simulink library "PS3Controller"  (R2026a)
settings: Solver=VariableStepAuto
settings Model: Creator=ebene  LastModifiedBy=ebene

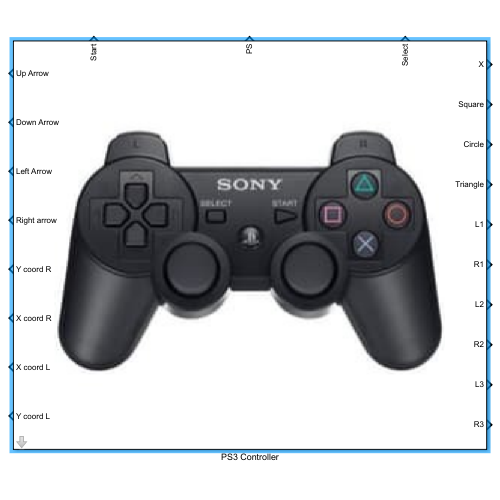
[thumbnail: Simulink's stored preview of the top-level diagram]
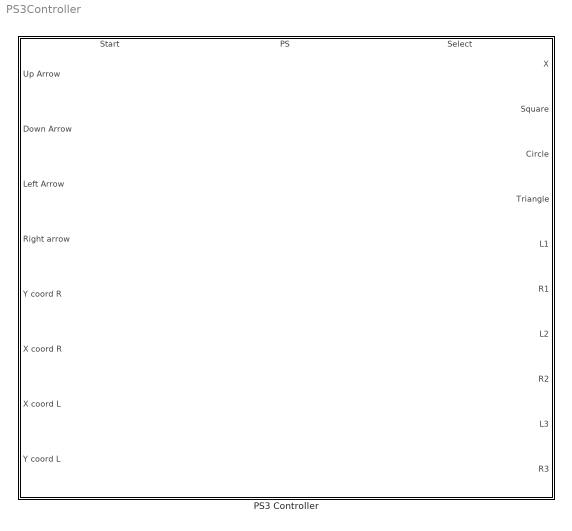
== system PS3Controller ==
  PS3 Controller : Subsystem  mask{SampleTime=0.01}
      settings: PortSchema="{\"entries\":[{\"content\":{\"sides\":[{\"content\":{\"connectorIds\":[\"Out14\",\"Out15\",\"Out16\",\"Out17\",\"Out18\",\"Out19\",\"Out20\",\"Out21\"]},\"type\":\"ConnectorPlacement.EquallySpacedRectSide\",\"uuid\":\"9967aca9-b04f-4513-919b-1d406207fdaf\"},{\"content\":{\"connectorIds\":[\"Out1\",\"Out2\",\"Out3\",\"Out4\",\"Out5\",\"Out6\",\"Out7\",\"Out8\",\"Out9\",\"Out10\"],\"side\":\"RIGHT\"},\"type\":\"ConnectorPlacement.EquallySpacedRectSide\",\"uuid\":\"a1d6af8d-11ae-4bef-92ba-22e763c87c3f\"},{\"content\":{\"connectorIds\":[\"Out11\",\"Out12\",\"Out13\"],\"side\":\"TOP\"},\"type\":\"ConnectorPlacement.EquallySpacedRectSide\",\"uuid\":\"54a133e6-d806-4ed2-95ca-5d9a3f88c0d3\"}]},\"type\":\"ConnectorPlacement.EquallySpacedConnector\",\"uuid\":\"1828c14f-a7e5-4350-a1b5-ffb3b45c04a4\"}],\"packageUris\":[\"http://schema.mathworks.com/mf0/Connector/R2020b\"],\"version\":\"1.0\"}"
      mask Display: image('PS3Controller.jpg', [10,10,10,10,100,100]);

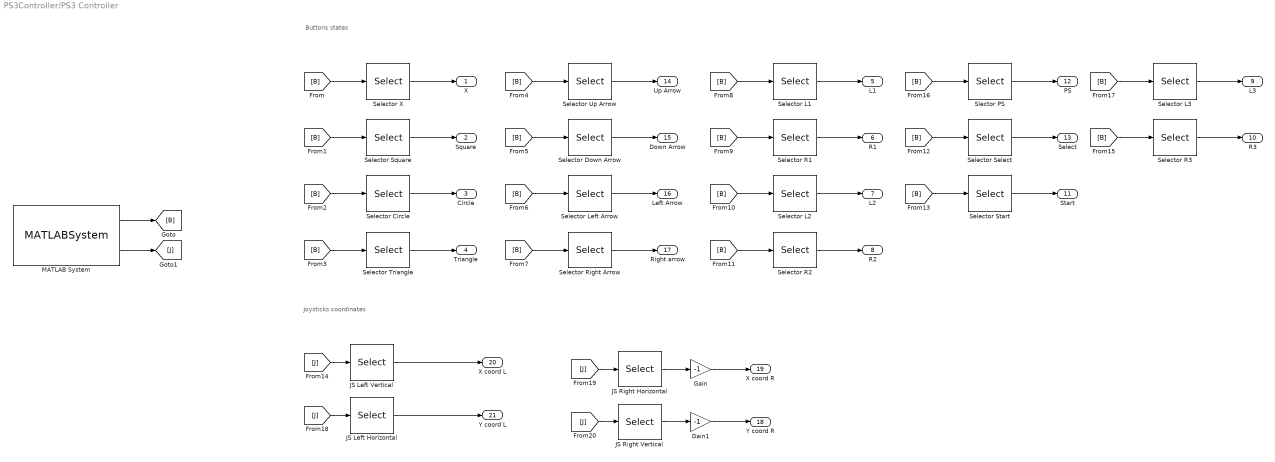
== system PS3Controller/PS3 Controller ==
  note: Joysticks coordinates
  note: Buttons states
  Gain : Gain  Gain=-1
  Gain1 : Gain  Gain=-1
  JS Left Horizontal : Selector  NumberOfDimensions=2  IndexMode=Zero-based  InputPortWidth=3  IndexOptions=Index vector (dialog),Index vector (dialog)  Indices=0,0  OutputSizes=1,1
  JS Left Vertical : Selector  NumberOfDimensions=2  IndexMode=Zero-based  InputPortWidth=3  IndexOptions=Index vector (dialog),Index vector (dialog)  Indices=0,1  OutputSizes=1,1
  JS Right Horizontal : Selector  NumberOfDimensions=2  IndexMode=Zero-based  InputPortWidth=3  IndexOptions=Index vector (dialog),Index vector (dialog)  Indices=0,3  OutputSizes=1,1
  JS Right Vertical : Selector  NumberOfDimensions=2  IndexMode=Zero-based  InputPortWidth=3  IndexOptions=Index vector (dialog),Index vector (dialog)  Indices=0,4  OutputSizes=1,1
  MATLAB System : MATLABSystem  System=PS3  SampleTime=SampleTime
      mask Type: PS3
  Selector Circle : Selector  NumberOfDimensions=2  IndexMode=Zero-based  InputPortWidth=3  IndexOptions=Index vector (dialog),Index vector (dialog)  Indices=0,1  OutputSizes=1,1
  Selector Down Arrow : Selector  NumberOfDimensions=2  IndexMode=Zero-based  InputPortWidth=3  IndexOptions=Index vector (dialog),Index vector (dialog)  Indices=0,14  OutputSizes=1,1
  Selector L1 : Selector  NumberOfDimensions=2  IndexMode=Zero-based  InputPortWidth=3  IndexOptions=Index vector (dialog),Index vector (dialog)  Indices=0,4  OutputSizes=1,1
  Selector L2 : Selector  NumberOfDimensions=2  IndexMode=Zero-based  InputPortWidth=3  IndexOptions=Index vector (dialog),Index vector (dialog)  Indices=0,6  OutputSizes=1,1
  Selector L3 : Selector  NumberOfDimensions=2  IndexMode=Zero-based  InputPortWidth=3  IndexOptions=Index vector (dialog),Index vector (dialog)  Indices=0,11  OutputSizes=1,1
  Selector Left Arrow : Selector  NumberOfDimensions=2  IndexMode=Zero-based  InputPortWidth=3  IndexOptions=Index vector (dialog),Index vector (dialog)  Indices=0,15  OutputSizes=1,1
  Selector R1 : Selector  NumberOfDimensions=2  IndexMode=Zero-based  InputPortWidth=3  IndexOptions=Index vector (dialog),Index vector (dialog)  Indices=0,5  OutputSizes=1,1
  Selector R2 : Selector  NumberOfDimensions=2  IndexMode=Zero-based  InputPortWidth=3  IndexOptions=Index vector (dialog),Index vector (dialog)  Indices=0,7  OutputSizes=1,1
  Selector R3 : Selector  NumberOfDimensions=2  IndexMode=Zero-based  InputPortWidth=3  IndexOptions=Index vector (dialog),Index vector (dialog)  Indices=0,12  OutputSizes=1,1
  Selector Right Arrow : Selector  NumberOfDimensions=2  IndexMode=Zero-based  InputPortWidth=3  IndexOptions=Index vector (dialog),Index vector (dialog)  Indices=0,16  OutputSizes=1,1
  Selector Select : Selector  NumberOfDimensions=2  IndexMode=Zero-based  InputPortWidth=3  IndexOptions=Index vector (dialog),Index vector (dialog)  Indices=0,8  OutputSizes=1,1
  Selector Square : Selector  NumberOfDimensions=2  IndexMode=Zero-based  InputPortWidth=3  IndexOptions=Index vector (dialog),Index vector (dialog)  Indices=0,3  OutputSizes=1,1
  Selector Start : Selector  NumberOfDimensions=2  IndexMode=Zero-based  InputPortWidth=3  IndexOptions=Index vector (dialog),Index vector (dialog)  Indices=0,9  OutputSizes=1,1
  Selector Triangle : Selector  NumberOfDimensions=2  IndexMode=Zero-based  InputPortWidth=3  IndexOptions=Index vector (dialog),Index vector (dialog)  Indices=0,2  OutputSizes=1,1
  Selector Up Arrow : Selector  NumberOfDimensions=2  IndexMode=Zero-based  InputPortWidth=3  IndexOptions=Index vector (dialog),Index vector (dialog)  Indices=0,13  OutputSizes=1,1
  Selector X : Selector  NumberOfDimensions=2  IndexMode=Zero-based  InputPortWidth=3  IndexOptions=Index vector (dialog),Index vector (dialog)  Indices=0,0  OutputSizes=1,1
  Slector PS : Selector  NumberOfDimensions=2  IndexMode=Zero-based  InputPortWidth=3  IndexOptions=Index vector (dialog),Index vector (dialog)  Indices=0,10  OutputSizes=1,1
  X : Outport
  Square : Outport  Port=2
  Circle : Outport  Port=3
  Triangle : Outport  Port=4
  L1 : Outport  Port=5
  R1 : Outport  Port=6
  L2 : Outport  Port=7
  R2 : Outport  Port=8
  L3 : Outport  Port=9
  R3 : Outport  Port=10
  Start : Outport  Port=11
  PS : Outport  Port=12
  Select : Outport  Port=13
  Up Arrow : Outport  Port=14
  Down Arrow : Outport  Port=15
  Left Arrow : Outport  Port=16
  Right arrow : Outport  Port=17
  Y coord R : Outport  Port=18
  X coord R : Outport  Port=19
  X coord L : Outport  Port=20
  Y coord L : Outport  Port=21
  wires:
  MATLAB System/1 -> [B]
  Selector R2/1 -> R2/1
  Selector L1/1 -> L1/1
  Selector Right Arrow/1 -> Right arrow/1
  [B] -> Selector R1/1
  Gain/1 -> X coord R/1
  [B] -> Selector Triangle/1
  [B] -> Selector X/1
  JS Left Vertical/1 -> X coord L/1
  JS Right Horizontal/1 -> Gain/1
  [B] -> Selector R3/1
  [B] -> Selector L2/1
  Selector X/1 -> X/1
  JS Right Vertical/1 -> Gain1/1
  Slector PS/1 -> PS/1
  [B] -> Slector PS/1
  [B] -> Selector Left Arrow/1
  Selector Select/1 -> Select/1
  Selector R1/1 -> R1/1
  [J] -> JS Right Horizontal/1
  Selector L2/1 -> L2/1
  JS Left Horizontal/1 -> Y coord L/1
  Selector Triangle/1 -> Triangle/1
  Selector Circle/1 -> Circle/1
  Selector R3/1 -> R3/1
  [B] -> Selector Select/1
  Selector Start/1 -> Start/1
  [B] -> Selector R2/1
  Selector Down Arrow/1 -> Down Arrow/1
  [B] -> Selector L1/1
  [B] -> Selector Start/1
  [B] -> Selector Circle/1
  Gain1/1 -> Y coord R/1
  [B] -> Selector Up Arrow/1
  MATLAB System/2 -> [J]
  [B] -> Selector Square/1
  Selector L3/1 -> L3/1
  [J] -> JS Right Vertical/1
  [J] -> JS Left Vertical/1
  [B] -> Selector Down Arrow/1
  Selector Square/1 -> Square/1
  Selector Up Arrow/1 -> Up Arrow/1
  [J] -> JS Left Horizontal/1
  Selector Left Arrow/1 -> Left Arrow/1
  [B] -> Selector L3/1
  [B] -> Selector Right Arrow/1
